simulink model "AEBSampleSimulink"  (Simulink 9.1)
settings: Solver=ode1  StartTime=0.0  StopTime=inf  FixedStep=0.001  RelTol=1e-3
undefined symbols (not defined in the file): azimuth_angle, DataStoreNumPara, elevation_angle, GroundTruth_Objects, heading, id, range_bbox, range_center, shape, time, type, velocity, width
(part 2 of 2)

== matlab function Veh_1/ComplexVehicleModel/RoadInfo/Subsystem/front_right ==
  data: out output double; xarry input double; yarray input double; zarray input double; dzdxarray input double; dzdyarray input double; muarray input double; x input double; y input double
function out  = fcn(xarry,yarray,zarray,dzdxarray,dzdyarray,muarray,x,y)
[x1,y1,x2,y2,x3,y3,x4,y4] = fcn_getpoint(xarry,yarray);
data_array = fcn_getdata(zarray,dzdxarray, dzdyarray,muarray);

zero = 0.001;
if ( abs(y2-y1) > zero )
   angle = 2*pi -  atan2(y2-y1,x2-x1);
   sin_angle = sin(angle);
   cos_angle = cos(angle);
   [x1,y1] = fcn_convert(x1,y1,x1,y1,sin_angle,cos_angle);
   [x2,y2] = fcn_convert(x1,y1,x2,y2,sin_angle,cos_angle);
   [x3,y3] = fcn_convert(x1,y1,x3,y3,sin_angle,cos_angle);
   [x4,y4] = fcn_convert(x1,y1,x4,y4,sin_angle,cos_angle);
   [x,y] = fcn_convert(x1,y1,x,y,sin_angle,cos_angle);
end

axle_x_left  = min(x1,x2);
axle_x_right = max(x1,x2);
axle_y_up    = max(y2,y3);
axle_y_down  = min(y2,y3);

% after rotota
% p1  p2
%
% p3 p4
z = 0;
dzdx = 0;
dzdy = 0;
mu = 0;
if ( x > axle_x_left ) && ( x < axle_x_right ) && ( y > axle_y_down ) && ( y < axle_y_up )
    xx1 = x3;
    xx2 = x4;
    yy1 = y3;
    yy2 = y1;
    matrix_left = [xx2-x  x-xx1];
    matrix_right = [ yy2 - y; y-yy1 ];
    delta = (xx2-xx1)*(yy2-yy1);
    delta = 1.0/delta;
    [z, dzdx, dzdy, mu] = fcn_cal(matrix_left,matrix_right,delta,data_array);
else
    if ( y >= axle_y_up ) 
        [z, dzdx, dzdy, mu] = fcn_cal_getmax(data_array(1,:),data_array(2,:));
    end
    if ( y <= axle_y_down )
        [z, dzdx, dzdy, mu] = fcn_cal_getmax(data_array(3,:),data_array(4,:));
    end
    if ( x >= axle_x_right )
        [z, dzdx, dzdy, mu] = fcn_cal_getmax(data_array(2,:),data_array(4,:));
    end
    if ( x <= axle_x_left )
        [z, dzdx, dzdy, mu] = fcn_cal_getmax(data_array(1,:),data_array(3,:));
    end
end

out = [z dzdx dzdy mu];
end

function [xxx,yyy] = fcn_convert(x0,y0,x1,y1,sin_agnle,cos_angle)
    xxx = (x1-x0)*cos_angle - (y1-y0)*sin_agnle + x0;
    yyy = (x1-x0)*sin_agnle + (y1-y0)*cos_angle + y0;
end

function [x1,y1,x2,y2,x3,y3,x4,y4] = fcn_getpoint(xarry,yarray)
    x1 = xarry(1);
    x2 = xarry(2);
    x3 = xarry(3);
    x4 = xarry(4);
    y1 = yarray(1);
    y2 = yarray(2);
    y3 = yarray(3);
    y4 = yarray(4);
end

function ret = fcn_getdata(zarray,dzdxarray, dzdyarray,muarray)
    ret = [ 
        zarray(1),dzdxarray(1),dzdyarray(1),muarray(1);
        zarray(2),dzdxarray(2),dzdyarray(2),muarray(2);
        zarray(3),dzdxarray(3),dzdyarray(3),muarray(3);
        zarray(4),dzdxarray(4),dzdyarray(4),muarray(4);
    ];
end

function [z,dzdx,dzdy,mu] = fcn_cal(matrix_left,matrix_right , delta, data_array)
%matrix_z = [z3, z1; z4 , z2]
%value = [xx2-x  x-xx1] * matrix * [ yy2 - y; y-yy1 ]  * d1
    array_z = data_array(:,1);
    array_dzdx = data_array(:,2);
    array_dzdy = data_array(:,3);
    array_mu = data_array(:,4);
    z = matrix_left * [array_z(3), array_z(1); array_z(4),array_z(2)] * matrix_right  * delta;
    dzdx = matrix_left * [array_dzdx(3), array_dzdx(1); array_dzdx(4),array_dzdx(2)] * matrix_right  * delta;
    dzdy = matrix_left * [array_dzdy(3), array_dzdy(1); array_dzdy(4),array_dzdy(2)] * matrix_right  * delta;
    mu = matrix_left * [array_mu(3), array_mu(1); array_mu(4),array_mu(2)] * matrix_right  * delta;
end

function [z,dzdx,dzdy,mu] = fcn_cal_getmax(data1,data2)
    z = max(data1(1),data2(1));
    dzdx = max(data1(2),data2(2));
    dzdy = max(data1(3),data2(3));
    mu = max(data1(4),data2(4));
end

== matlab function Veh_1/ComplexVehicleModel/RoadInfo/Subsystem/front_left ==
  data: out output double; xarry input double; yarray input double; zarray input double; dzdxarray input double; dzdyarray input double; muarray input double; x input double; y input double
function out  = fcn(xarry,yarray,zarray,dzdxarray,dzdyarray,muarray,x,y)
[x1,y1,x2,y2,x3,y3,x4,y4] = fcn_getpoint(xarry,yarray);
data_array = fcn_getdata(zarray,dzdxarray, dzdyarray,muarray);

zero = 0.001;
if ( abs(y2-y1) > zero )
   angle = 2*pi -  atan2(y2-y1,x2-x1);
   sin_angle = sin(angle);
   cos_angle = cos(angle);
   [x1,y1] = fcn_convert(x1,y1,x1,y1,sin_angle,cos_angle);
   [x2,y2] = fcn_convert(x1,y1,x2,y2,sin_angle,cos_angle);
   [x3,y3] = fcn_convert(x1,y1,x3,y3,sin_angle,cos_angle);
   [x4,y4] = fcn_convert(x1,y1,x4,y4,sin_angle,cos_angle);
   [x,y] = fcn_convert(x1,y1,x,y,sin_angle,cos_angle);
end

axle_x_left  = min(x1,x2);
axle_x_right = max(x1,x2);
axle_y_up    = max(y2,y3);
axle_y_down  = min(y2,y3);

% after rotota
% p1  p2
%
% p3 p4
z = 0;
dzdx = 0;
dzdy = 0;
mu = 0;
if ( x > axle_x_left ) && ( x < axle_x_right ) && ( y > axle_y_down ) && ( y < axle_y_up )
    xx1 = x3;
    xx2 = x4;
    yy1 = y3;
    yy2 = y1;
    matrix_left = [xx2-x  x-xx1];
    matrix_right = [ yy2 - y; y-yy1 ];
    delta = (xx2-xx1)*(yy2-yy1);
    delta = 1.0/delta;
    [z, dzdx, dzdy, mu] = fcn_cal(matrix_left,matrix_right,delta,data_array);
else
    if ( y >= axle_y_up ) 
        [z, dzdx, dzdy, mu] = fcn_cal_getmax(data_array(1,:),data_array(2,:));
    end
    if ( y <= axle_y_down )
        [z, dzdx, dzdy, mu] = fcn_cal_getmax(data_array(3,:),data_array(4,:));
    end
    if ( x >= axle_x_right )
        [z, dzdx, dzdy, mu] = fcn_cal_getmax(data_array(2,:),data_array(4,:));
    end
    if ( x <= axle_x_left )
        [z, dzdx, dzdy, mu] = fcn_cal_getmax(data_array(1,:),data_array(3,:));
    end
end

out = [z dzdx dzdy mu];
end

function [xxx,yyy] = fcn_convert(x0,y0,x1,y1,sin_agnle,cos_angle)
    xxx = (x1-x0)*cos_angle - (y1-y0)*sin_agnle + x0;
    yyy = (x1-x0)*sin_agnle + (y1-y0)*cos_angle + y0;
end

function [x1,y1,x2,y2,x3,y3,x4,y4] = fcn_getpoint(xarry,yarray)
    x1 = xarry(1);
    x2 = xarry(2);
    x3 = xarry(3);
    x4 = xarry(4);
    y1 = yarray(1);
    y2 = yarray(2);
    y3 = yarray(3);
    y4 = yarray(4);
end

function ret = fcn_getdata(zarray,dzdxarray, dzdyarray,muarray)
    ret = [ 
        zarray(1),dzdxarray(1),dzdyarray(1),muarray(1);
        zarray(2),dzdxarray(2),dzdyarray(2),muarray(2);
        zarray(3),dzdxarray(3),dzdyarray(3),muarray(3);
        zarray(4),dzdxarray(4),dzdyarray(4),muarray(4);
    ];
end

function [z,dzdx,dzdy,mu] = fcn_cal(matrix_left,matrix_right , delta, data_array)
%matrix_z = [z3, z1; z4 , z2]
%value = [xx2-x  x-xx1] * matrix * [ yy2 - y; y-yy1 ]  * d1
    array_z = data_array(:,1);
    array_dzdx = data_array(:,2);
    array_dzdy = data_array(:,3);
    array_mu = data_array(:,4);
    z = matrix_left * [array_z(3), array_z(1); array_z(4),array_z(2)] * matrix_right  * delta;
    dzdx = matrix_left * [array_dzdx(3), array_dzdx(1); array_dzdx(4),array_dzdx(2)] * matrix_right  * delta;
    dzdy = matrix_left * [array_dzdy(3), array_dzdy(1); array_dzdy(4),array_dzdy(2)] * matrix_right  * delta;
    mu = matrix_left * [array_mu(3), array_mu(1); array_mu(4),array_mu(2)] * matrix_right  * delta;
end

function [z,dzdx,dzdy,mu] = fcn_cal_getmax(data1,data2)
    z = max(data1(1),data2(1));
    dzdx = max(data1(2),data2(2));
    dzdy = max(data1(3),data2(3));
    mu = max(data1(4),data2(4));
end

== matlab function Veh_1/ComplexVehicleModel/RoadInfo/Subsystem/tail_left ==
  data: out output double; xarry input double; yarray input double; zarray input double; dzdxarray input double; dzdyarray input double; muarray input double; x input double; y input double
function out  = fcn(xarry,yarray,zarray,dzdxarray,dzdyarray,muarray,x,y)
[x1,y1,x2,y2,x3,y3,x4,y4] = fcn_getpoint(xarry,yarray);
data_array = fcn_getdata(zarray,dzdxarray, dzdyarray,muarray);

zero = 0.001;
if ( abs(y2-y1) > zero )
   angle = 2*pi -  atan2(y2-y1,x2-x1);
   sin_angle = sin(angle);
   cos_angle = cos(angle);
   [x1,y1] = fcn_convert(x1,y1,x1,y1,sin_angle,cos_angle);
   [x2,y2] = fcn_convert(x1,y1,x2,y2,sin_angle,cos_angle);
   [x3,y3] = fcn_convert(x1,y1,x3,y3,sin_angle,cos_angle);
   [x4,y4] = fcn_convert(x1,y1,x4,y4,sin_angle,cos_angle);
   [x,y] = fcn_convert(x1,y1,x,y,sin_angle,cos_angle);
end

axle_x_left  = min(x1,x2);
axle_x_right = max(x1,x2);
axle_y_up    = max(y2,y3);
axle_y_down  = min(y2,y3);

% after rotota
% p1  p2
%
% p3 p4
z = 0;
dzdx = 0;
dzdy = 0;
mu = 0;
if ( x > axle_x_left ) && ( x < axle_x_right ) && ( y > axle_y_down ) && ( y < axle_y_up )
    xx1 = x3;
    xx2 = x4;
    yy1 = y3;
    yy2 = y1;
    matrix_left = [xx2-x  x-xx1];
    matrix_right = [ yy2 - y; y-yy1 ];
    delta = (xx2-xx1)*(yy2-yy1);
    delta = 1.0/delta;
    [z, dzdx, dzdy, mu] = fcn_cal(matrix_left,matrix_right,delta,data_array);
else
    if ( y >= axle_y_up ) 
        [z, dzdx, dzdy, mu] = fcn_cal_getmax(data_array(1,:),data_array(2,:));
    end
    if ( y <= axle_y_down )
        [z, dzdx, dzdy, mu] = fcn_cal_getmax(data_array(3,:),data_array(4,:));
    end
    if ( x >= axle_x_right )
        [z, dzdx, dzdy, mu] = fcn_cal_getmax(data_array(2,:),data_array(4,:));
    end
    if ( x <= axle_x_left )
        [z, dzdx, dzdy, mu] = fcn_cal_getmax(data_array(1,:),data_array(3,:));
    end
end

out = [z dzdx dzdy mu];
end

function [xxx,yyy] = fcn_convert(x0,y0,x1,y1,sin_agnle,cos_angle)
    xxx = (x1-x0)*cos_angle - (y1-y0)*sin_agnle + x0;
    yyy = (x1-x0)*sin_agnle + (y1-y0)*cos_angle + y0;
end

function [x1,y1,x2,y2,x3,y3,x4,y4] = fcn_getpoint(xarry,yarray)
    x1 = xarry(1);
    x2 = xarry(2);
    x3 = xarry(3);
    x4 = xarry(4);
    y1 = yarray(1);
    y2 = yarray(2);
    y3 = yarray(3);
    y4 = yarray(4);
end

function ret = fcn_getdata(zarray,dzdxarray, dzdyarray,muarray)
    ret = [ 
        zarray(1),dzdxarray(1),dzdyarray(1),muarray(1);
        zarray(2),dzdxarray(2),dzdyarray(2),muarray(2);
        zarray(3),dzdxarray(3),dzdyarray(3),muarray(3);
        zarray(4),dzdxarray(4),dzdyarray(4),muarray(4);
    ];
end

function [z,dzdx,dzdy,mu] = fcn_cal(matrix_left,matrix_right , delta, data_array)
%matrix_z = [z3, z1; z4 , z2]
%value = [xx2-x  x-xx1] * matrix * [ yy2 - y; y-yy1 ]  * d1
    array_z = data_array(:,1);
    array_dzdx = data_array(:,2);
    array_dzdy = data_array(:,3);
    array_mu = data_array(:,4);
    z = matrix_left * [array_z(3), array_z(1); array_z(4),array_z(2)] * matrix_right  * delta;
    dzdx = matrix_left * [array_dzdx(3), array_dzdx(1); array_dzdx(4),array_dzdx(2)] * matrix_right  * delta;
    dzdy = matrix_left * [array_dzdy(3), array_dzdy(1); array_dzdy(4),array_dzdy(2)] * matrix_right  * delta;
    mu = matrix_left * [array_mu(3), array_mu(1); array_mu(4),array_mu(2)] * matrix_right  * delta;
end

function [z,dzdx,dzdy,mu] = fcn_cal_getmax(data1,data2)
    z = max(data1(1),data2(1));
    dzdx = max(data1(2),data2(2));
    dzdy = max(data1(3),data2(3));
    mu = max(data1(4),data2(4));
end

== matlab function Veh_1/ComplexVehicleModel/RoadInfo/Subsystem/tail_right ==
  data: out output double; xarry input double; yarray input double; zarray input double; dzdxarray input double; dzdyarray input double; muarray input double; x input double; y input double
function out  = fcn(xarry,yarray,zarray,dzdxarray,dzdyarray,muarray,x,y)
[x1,y1,x2,y2,x3,y3,x4,y4] = fcn_getpoint(xarry,yarray);
data_array = fcn_getdata(zarray,dzdxarray, dzdyarray,muarray);

zero = 0.001;
if ( abs(y2-y1) > zero )
   angle = 2*pi -  atan2(y2-y1,x2-x1);
   sin_angle = sin(angle);
   cos_angle = cos(angle);
   [x1,y1] = fcn_convert(x1,y1,x1,y1,sin_angle,cos_angle);
   [x2,y2] = fcn_convert(x1,y1,x2,y2,sin_angle,cos_angle);
   [x3,y3] = fcn_convert(x1,y1,x3,y3,sin_angle,cos_angle);
   [x4,y4] = fcn_convert(x1,y1,x4,y4,sin_angle,cos_angle);
   [x,y] = fcn_convert(x1,y1,x,y,sin_angle,cos_angle);
end

axle_x_left  = min(x1,x2);
axle_x_right = max(x1,x2);
axle_y_up    = max(y2,y3);
axle_y_down  = min(y2,y3);

% after rotota
% p1  p2
%
% p3 p4
z = 0;
dzdx = 0;
dzdy = 0;
mu = 0;
if ( x > axle_x_left ) && ( x < axle_x_right ) && ( y > axle_y_down ) && ( y < axle_y_up )
    xx1 = x3;
    xx2 = x4;
    yy1 = y3;
    yy2 = y1;
    matrix_left = [xx2-x  x-xx1];
    matrix_right = [ yy2 - y; y-yy1 ];
    delta = (xx2-xx1)*(yy2-yy1);
    delta = 1.0/delta;
    [z, dzdx, dzdy, mu] = fcn_cal(matrix_left,matrix_right,delta,data_array);
else
    if ( y >= axle_y_up ) 
        [z, dzdx, dzdy, mu] = fcn_cal_getmax(data_array(1,:),data_array(2,:));
    end
    if ( y <= axle_y_down )
        [z, dzdx, dzdy, mu] = fcn_cal_getmax(data_array(3,:),data_array(4,:));
    end
    if ( x >= axle_x_right )
        [z, dzdx, dzdy, mu] = fcn_cal_getmax(data_array(2,:),data_array(4,:));
    end
    if ( x <= axle_x_left )
        [z, dzdx, dzdy, mu] = fcn_cal_getmax(data_array(1,:),data_array(3,:));
    end
end

out = [z dzdx dzdy mu];
end

function [xxx,yyy] = fcn_convert(x0,y0,x1,y1,sin_agnle,cos_angle)
    xxx = (x1-x0)*cos_angle - (y1-y0)*sin_agnle + x0;
    yyy = (x1-x0)*sin_agnle + (y1-y0)*cos_angle + y0;
end

function [x1,y1,x2,y2,x3,y3,x4,y4] = fcn_getpoint(xarry,yarray)
    x1 = xarry(1);
    x2 = xarry(2);
    x3 = xarry(3);
    x4 = xarry(4);
    y1 = yarray(1);
    y2 = yarray(2);
    y3 = yarray(3);
    y4 = yarray(4);
end

function ret = fcn_getdata(zarray,dzdxarray, dzdyarray,muarray)
    ret = [ 
        zarray(1),dzdxarray(1),dzdyarray(1),muarray(1);
        zarray(2),dzdxarray(2),dzdyarray(2),muarray(2);
        zarray(3),dzdxarray(3),dzdyarray(3),muarray(3);
        zarray(4),dzdxarray(4),dzdyarray(4),muarray(4);
    ];
end

function [z,dzdx,dzdy,mu] = fcn_cal(matrix_left,matrix_right , delta, data_array)
%matrix_z = [z3, z1; z4 , z2]
%value = [xx2-x  x-xx1] * matrix * [ yy2 - y; y-yy1 ]  * d1
    array_z = data_array(:,1);
    array_dzdx = data_array(:,2);
    array_dzdy = data_array(:,3);
    array_mu = data_array(:,4);
    z = matrix_left * [array_z(3), array_z(1); array_z(4),array_z(2)] * matrix_right  * delta;
    dzdx = matrix_left * [array_dzdx(3), array_dzdx(1); array_dzdx(4),array_dzdx(2)] * matrix_right  * delta;
    dzdy = matrix_left * [array_dzdy(3), array_dzdy(1); array_dzdy(4),array_dzdy(2)] * matrix_right  * delta;
    mu = matrix_left * [array_mu(3), array_mu(1); array_mu(4),array_mu(2)] * matrix_right  * delta;
end

function [z,dzdx,dzdy,mu] = fcn_cal_getmax(data1,data2)
    z = max(data1(1),data2(1));
    dzdx = max(data1(2),data2(2));
    dzdy = max(data1(3),data2(3));
    mu = max(data1(4),data2(4));
end

== matlab function Veh_1/ComplexVehicleModel/RoadInfo/Subsystem/front_right1 ==
  data: z output double; fl input double; fr input double; tl input double; tr input double; dzdx output double; dzdy output double; mu output double
function [z,dzdx,dzdy,mu]  = fcn(fl,fr,tl,tr)
    z =  [fl(1),fr(1),tl(1),tr(1)];
    dzdx = [fl(2),fr(2),tl(2),tr(2)];
    dzdy = [fl(3),fr(3),tl(3),tr(3)];
    mu =   [fl(4),fr(4),tl(4),tr(4)];
end

== matlab function Veh_1/ComplexVehicleModel/RoadInfo/Subsystem1/front_right ==
  data: p1 output double; array1 input double; array2 input double; p2 output double; p3 output double; p4 output double
function [p1,p2,p3,p4]  = fcn(array1,array2)
    p1 = [array1(1),array2(1)];
    p2 = [array1(2),array2(2)];
    p3 = [array1(3),array2(3)];
    p4 = [array1(4),array2(4)];
end

== matlab function Veh_1/ComplexVehicleModel/RoadInfo/Subsystem/Cal_Height ==
  data: retHeight output double; bumsNum input double; x1array input double; y1array input double; x2array input double; y2array input double; x3array input double; y3array input double; x4array input double; y4array input double; heightarray input double; px0 input double; py0 input double; px1 input double; py1 input double; px2 input double; py2 input double; px3 input double; py3 input double; retValue output double
function [retHeight,retValue]   = fcn(bumsNum,x1array,y1array,x2array,y2array,x3array,y3array,x4array,y4array,heightarray,px0,py0,px1,py1,px2,py2,px3,py3)
h0 = 0.0;
h1 = 0.0;
h2 = 0.0;
h3 = 0.0;
value0 = 0;
value1 = 0;
value2 = 0;
value3 = 0;
for index = 1:bumsNum+1
     v = fcn_in_sqar(x1array(index),y1array(index),x2array(index),y2array(index),x3array(index),y3array(index),x4array(index),y4array(index),px0,py0);
     if (v > 0)
         value0 = 1;
         h0 =  heightarray(index);
         break;
     end
end
for index = 1:bumsNum+1
     v = fcn_in_sqar(x1array(index),y1array(index),x2array(index),y2array(index),x3array(index),y3array(index),x4array(index),y4array(index),px1,py1);
     if (v > 0)
         value1 = 1;
         h1 =  heightarray(index);
         break;
     end
end

for index = 1:bumsNum+1
     v = fcn_in_sqar(x1array(index),y1array(index),x2array(index),y2array(index),x3array(index),y3array(index),x4array(index),y4array(index),px2,py2);
     if (v > 0)
         value2 = 1;
         h2 =  heightarray(index);
         break;
     end
end

for index = 1:bumsNum+1
     v = fcn_in_sqar(x1array(index),y1array(index),x2array(index),y2array(index),x3array(index),y3array(index),x4array(index),y4array(index),px3,py3);
     if (v > 0)
         value3 = 1;
         h3 =  heightarray(index);
         break;
     end
end
retHeight = [h0,h1,h2,h3];
retValue = [value0,value1,value2,value3];
end


function ret = fcn_in_sqar(x1,y1,x2,y2,x3,y3,x4,y4,x,y)
    ret = 0;
    a = (x2-x1)*(y-y1)-(y2-y1)*(x-x1);
    b = (x3-x2)*(y-y2)-(y3-y2)*(x-x2);
    c = (x4-x3)*(y-y3)-(y4-y3)*(x-x3);
    d = (x1-x4)*(y-y4)-(y1-y4)*(x-x4);
    if (a>=0&&b>=0&&c>=0&&d>=0)
        ret = 1;
    end
    if (a<=0&&b<=0&&c<=0&&d<=0)
        ret = 1;
    end
end

== matlab function Veh_1/ComplexVehicleModel/RoadInfo/Subsystem/AddHeight ==
  data: z output double; height input double; roadZ input double
function z  = fcn(height,roadZ)
    z =  [roadZ(1)+height(1),roadZ(2)+height(2),roadZ(3)+height(3),roadZ(4)+height(4)];
end

== matlab function Veh_1/Algorithm/ControlSignalFilter/MATLAB Function ==
  data: driver input double; valid output double; algoThrottle input double; algoBrake input double; algoSteer input double; algoMode input double; algoGear input double; throttle output double; brake output double; steer output double; mode output double; gear output double
function [valid,throttle,brake,steer,mode,gear] = fcn(driver,algoThrottle,algoBrake,algoSteer,algoMode,algoGear)
valid = driver(1) + algoThrottle(2) + algoBrake(2) + algoSteer(2) + algoMode(2) + algoGear(2);
if valid > 0
    valid = 1;
end

throttle = fcnValidData(driver(2),algoThrottle(3),algoThrottle(2));
brake = fcnValidData(driver(3),algoBrake(3),algoBrake(2));
steer = fcnValidData(driver(4),algoSteer(3),algoSteer(2));
mode = fcnValidData(driver(5),algoMode(3),algoMode(2));
gear = fcnValidData(driver(6),algoGear(3),algoGear(2));

end

function out = fcnValidData(data1,data2,valid)
    if valid > 0.5
        out = data2;
    else
        out = data1;
    end
end

== matlab function Veh_1/ComplexVehicleModel/RoadInfo/MATLAB Function ==
  data: fl input double; tire_x output double; fr input double; rl input double; rr input double; tire_y output double; tire_z output double
function [tire_x,tire_y,tire_z] = fcn(fl,fr,rl,rr)

tire_x = [fl(11),fr(11),rl(11),rr(11)];
tire_y = [fl(12),fr(12),rl(12),rr(12)];
tire_z = [fl(13),fr(13),rl(13),rr(13)];

== matlab function Veh_1/ComplexVehicleModel/RoadInfo/MATLAB Function1 ==
  data: t input double; outz output double; z input double; dzdx input double; dzdy input double; mu input double; tirez input double; outdzdx output double; outdzdy output double; outmu output double
function [outz,outdzdx,outdzdy,outmu] = fcn(t,z,dzdx,dzdy,mu,tirez)
%#codegen
outz = tirez;
outdzdx = [0,0,0,0];
outdzdy = [0,0,0,0];
outmu = [0.75,0.75,0.75,0.75];
if t > 0.001
    outz = z;
    outdzdx = dzdx;
    outdzdy = dzdy;
    outmu = mu;
end

== matlab function Veh_1/VehicleDataBus/MATLAB Function ==
  data: u input double; head output double; c_x output double; c_y output double; c_z output double; yaw output double; pitch output double; roll output double; rot_spd output double; f_x output double; f_y output double; f_z output double; g_x output double; g_y output double; g_z output double
function [head,c_x,c_y,c_z,yaw,pitch,roll,rot_spd,f_x,f_y,f_z,g_x,g_y,g_z] = fcn(u)
head = [u(1),u(2),u(3),u(4),u(5)];
start = 6;
c_x =   [u(start),u(start+13),u(start+26),u(start+39)];
start = 7;
c_y =   [u(start),u(start+13),u(start+26),u(start+39)];
start = 8;
c_z =   [u(start),u(start+13),u(start+26),u(start+39)];
start = 9;
yaw =   [u(start),u(start+13),u(start+26),u(start+39)];
start = 10;
pitch = [u(start),u(start+13),u(start+26),u(start+39)];
start = 11;
roll =  [u(start),u(start+13),u(start+26),u(start+39)];
start = 12;
rot_spd =  [u(start),u(start+13),u(start+26),u(start+39)];
start = 13;
f_x =  [u(start),u(start+13),u(start+26),u(start+39)];
start = 14;
f_y =  [u(start),u(start+13),u(start+26),u(start+39)];
start = 15;
f_z =  [u(start),u(start+13),u(start+26),u(start+39)];
start = 16;
g_x =  [u(start),u(start+13),u(start+26),u(start+39)];
start = 17;
g_y =  [u(start),u(start+13),u(start+26),u(start+39)];
start = 18;
g_z =  [u(start),u(start+13),u(start+26),u(start+39)];

== matlab function Veh_1/ComplexVehicleModel/MATLAB Function1 ==
  data: u input double; ego output double; egoextra output double
function [ego,egoextra] = fcn(u)

ego = [u(2),u(3),u(4),u(5),u(6),u(7),u(8)];
egoextra = [u(8),u(9),u(10),u(11),u(12),u(13),u(14),u(15),u(16),u(17),u(18),u(19)];

== matlab function Veh_1/ComplexVehicleModel/MATLAB Function2 ==
  data: driverControl input double; throttle output double; dynamicControl input double; brake output double; steer output double; mode output double
function [throttle,brake,steer,mode] = fcn(driverControl,dynamicControl)
%#codegen
if driverControl(1) > 0.5
    throttle = driverControl(2);
    brake = driverControl(3)* 1e6;
    steer = driverControl(4) * 0.0174;
    mode = driverControl(5);
else
    throttle = dynamicControl(3);
    brake = dynamicControl(4);
    steer = dynamicControl(5);
    mode = dynamicControl(2);
end

if mode > 0.5
   mode = 1 ;
end

== matlab function Veh_1/Algorithm/AEB Controller/MATLAB Function1 ==
  data: aeb_status input double; fcw_status input double; y output double
function y = fcn(aeb_status, fcw_status)
ret = 0;
if fcw_status > 0
   ret = 100;
end

if aeb_status > 0
    ret = 103;
end

if fcw_status > 0 && aeb_status > 0
    ret = 103;
end

y = cast(ret,'double');

== matlab function Veh_1/Algorithm/AEB Logical/Find Leader Car ==
  data: EGOX input double; RelatedDistance output double; EGOY input double; EGOV input double; EGOYAW input double; time input double; width input double; ids input double; types input double; shapes input double; range_centers input double; range_bboxs input double; azimuth_angles input double; elevation_angles input double; velocitys input double; headings input double; RelatedSpeed output double
function [RelatedDistance, RelatedSpeed]  = DetectionConcatenation(EGOX,EGOY,EGOV, EGOYAW, time, width, ids, types, shapes, range_centers, range_bboxs, azimuth_angles, elevation_angles, velocitys, headings)


% This function finds the lead car: a car in front of the ego car that
% satisfies all the criteria below:
% * Within the ego car's lane.
% * In front of the ego car.
% * Closest to the ego car.


% 1. The lane is defined using a parabolic model, where y=ax^2+bx+c. a is
%    equal to half the road curvature, b=0, and c is the offset of the lane
%    boundaries relative to the ego car. Overall lane width is assumed to
%    be 3.6m, typical highway lane width.
laneWidth = 3.6;

% 2. The ego car is assumed to be traveling in the middle of its lane, with
%    1.8m on each side of it. So, c=+1.8m for the left lane boundary and
%    -1.8m for the right lane boundary.
halfLaneWidth = laneWidth/2;

maxX = cast(500.0,'double');
Selected = cast(-1,'int32');

if(width > 0)
    for i = 1:width
        dis = range_bboxs(i);
        speed = velocitys(i);
        angle = -azimuth_angles(i);
        yaw = 3.1415926/2 - headings(i);
        deltaYaw = yaw - EGOYAW;
        x = dis * cos(angle); % Longitudinal position of the track relative to ego
        y = dis * sin(angle); % Lateral position of the track relative to ego
        if dis < maxX && dis > 0
            yleftLane  = polyval([0, 0,  halfLaneWidth],x); % Half a lane to the left
            yrightLane = polyval([0, 0, -halfLaneWidth],x); % Half a lane to the right

            % Find a new lead car
            if(yrightLane <= y) && (y<=yleftLane)
                maxX = cast(dis,'double');
                Selected = i;
            end
        end
    end
end

if(Selected ~= -1)
    RelatedDistance = cast(range_bboxs(Selected),'double');
    yaw = 3.1415926/2 - headings(Selected);
    speed = velocitys(Selected);
    deltaYaw = yaw - EGOYAW;
    Vxx = speed * cos(deltaYaw);
    %Vyy = speed * sin(deltaYaw);
    RelatedSpeed = cast(-EGOV + Vxx,'double');
else
    RelatedDistance = 500;
    RelatedSpeed = 0.1;
end

== matlab function Veh_1/Algorithm/AEB Controller/MATLAB Function ==
  data: u input double; y output double
function y = fcn(u)
persistent aeb_enable;
if isempty(aeb_enable)
    aeb_enable = 0;
end

if u > 0
    aeb_enable = 1;
else
    aeb_enable = 0;
end

if aeb_enable == 0
    y = 0;
else
    y = 1;
end

== stateflow chart Veh_1/Algorithm/AEB Controller/AEB Controller1/Braking Controller/AEBLogic ==
  note: FCW/AEB Logic
  state Default
    entry: AEBstatus = 0;
    FCWactivate = 0;
    decel = 0;
  state FCW
    entry: AEBstatus = 0;
    FCWactivate = 1;
    decel = 0;
  state Partial_Braking1
    entry: AEBstatus = 1;
    FCWactivate = 1;
    decel = PB1decel;
  state Full_Braking
    entry: AEBstatus = 3;
    FCWactivate = 1;
    decel = FBdecel;
  state Partial_Braking2
    entry: AEBstatus = 2;
    FCWactivate = 1;
    decel = PB2decel;
  (default) -> Default
  Full_Braking -> Default : [stop==1]
  Partial_Braking2 -> Default [order 2] : [stop==1]
  Partial_Braking1 -> Default [order 2] : [stop==1]
  Default -> FCW : [(abs(TTC)<FCWtime) && TTC<0]
  FCW -> Default [order 2] : [abs(TTC)>=1.2*FCWtime]
  FCW -> Partial_Braking1 [order 1] : [(abs(TTC) < PB1time) && TTC<0]
  Partial_Braking1 -> Partial_Braking2 [order 1] : [(abs(TTC) < PB2time) && TTC<0]
  Partial_Braking2 -> Full_Braking [order 1] : [(abs(TTC) < FBtime) && TTC<0]
  data: FCWactivate output uint8; TTC input double; FCWtime input double; PB1time input double; PB2time input double; FBtime input double; PB1decel input double; PB2decel input double; FBdecel input double; AEBstatus output uint8; decel output double; stop input double
